simulink model "ModeloBalancin"  (R2024a)
settings: Solver=VariableStepAuto  StartTime=0.0  StopTime=10.0  RelTol=1e-3
undefined symbols (not defined in the file): betaF, g, J, Kf, Lb1, Lb2, Lm, m_m, mb1, mb2
settings Model: Creator=Cami  LastModifiedBy=alfar

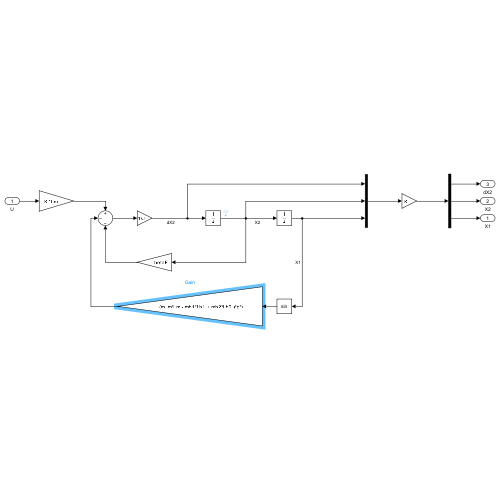
[thumbnail: Simulink's stored preview of the top-level diagram]
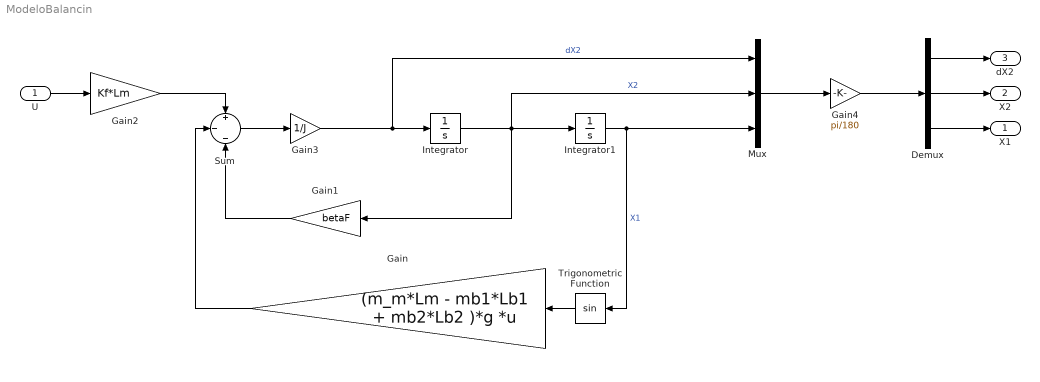
== system ModeloBalancin ==
  U : Inport
  Demux : Demux  Outputs=3
  Gain : Gain  Gain=(m_m*Lm - mb1*Lb1 + mb2*Lb2 )*g  Multiplication=Matrix(K*u)
  Gain1 : Gain  Gain=betaF
  Gain2 : Gain  Gain=Kf*Lm
  Gain3 : Gain  Gain=1/J
  Gain4 : Gain  Gain=pi/180
  Integrator : Integrator
  Integrator1 : Integrator
  Mux : Mux  Inputs=3
  Sum : Sum  Inputs=+|-|-
  Trigonometric Function : Trigonometry
  X1 : Outport
  X2 : Outport  Port=2
  dX2 : Outport  Port=3
  wires:
  Sum/1 -> Gain3/1
  Trigonometric Function/1 -> Gain/1
  Integrator/1 -> Mux/2, Gain1/1, Integrator1/1  "X2"
  Integrator1/1 -> Trigonometric Function/1, Mux/3  "X1"
  Gain2/1 -> Sum/1
  U/1 -> Gain2/1
  Gain1/1 -> Sum/3
  Gain/1 -> Sum/2
  Mux/1 -> Gain4/1
  Gain4/1 -> Demux/1
  Demux/2 -> X2/1
  Demux/1 -> dX2/1
  Demux/3 -> X1/1
  Gain3/1 -> Mux/1, Integrator/1  "dX2"
